simulink subsystem "POWER_GAIN"  (R2023a)
settings: Solver=VariableStepAuto  StartTime=0.0  StopTime=10.0  RelTol=1e-3
settings Model: Creator=hidra  LastModifiedBy=hidra

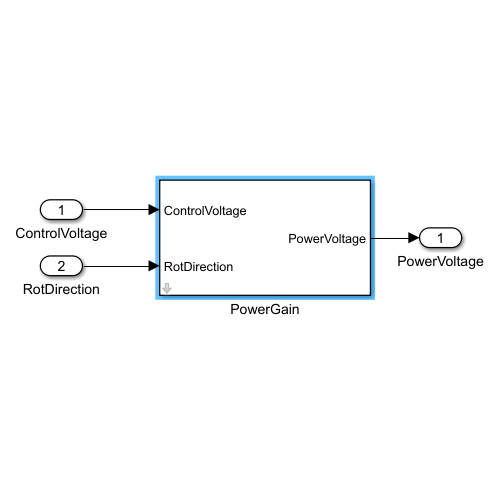
[thumbnail: Simulink's stored preview of the top-level diagram]
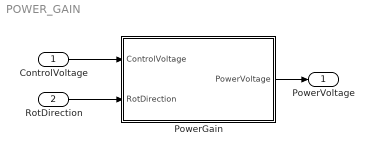
== system POWER_GAIN ==
  ControlVoltage : Inport
  RotDirection : Inport  Port=2
  PowerGain : Subsystem  mask{k=24/3.3, s=24}
      mask prompts: k "Gain"; s "Saturation"
  PowerVoltage : Outport
  wires:
  PowerGain/1(PowerVoltage) -> PowerVoltage/1
  ControlVoltage/1 -> PowerGain/1(ControlVoltage)
  RotDirection/1 -> PowerGain/2(RotDirection)

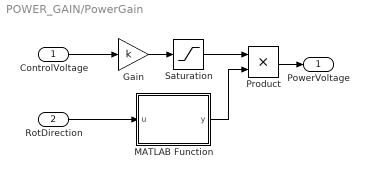
== system POWER_GAIN/PowerGain ==
  ControlVoltage : Inport
  RotDirection : Inport  Port=2
  Gain : Gain  Gain=k
  MATLAB Function : MATLAB Function  TreatAsAtomicUnit=on
  Product : Product
  Saturation : Saturate  UpperLimit=s  LowerLimit=0
  PowerVoltage : Outport
  wires:
  ControlVoltage/1 -> Gain/1
  MATLAB Function/1(y) -> Product/2
  Product/1 -> PowerVoltage/1
  Gain/1 -> Saturation/1
  RotDirection/1 -> MATLAB Function/1(u)
  Saturation/1 -> Product/1

== matlab function POWER_GAIN/PowerGain/MATLAB Function ==
  data: u input; y output
function y = fcn(u)
y = 1
if u == false;
y = -1;
end
